simulink model "transientStability_R2013B_MDL"  (Simulink 8.2)
settings: Solver=ode4  SolverMode=SingleTasking  StartTime=0.0  StopTime=10  FixedStep=0.01  MaxStep=0.01  RelTol=1e-3  AbsTol=1e-2
undefined symbols (not defined in the file): j, mpc
(part 4 of 4)

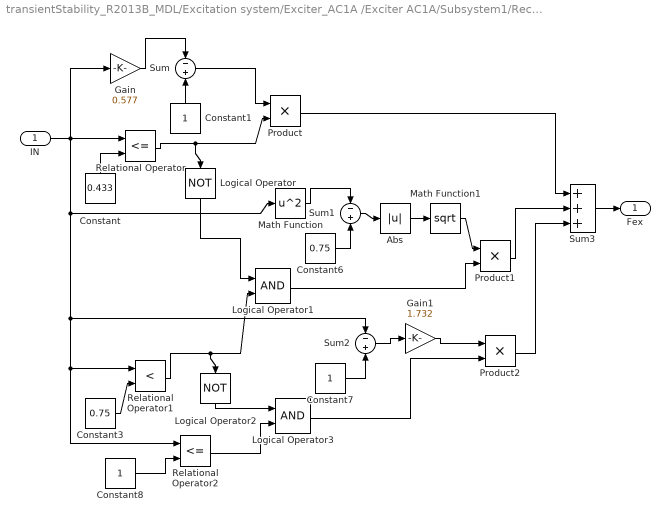
== system transientStability_R2013B_MDL/Excitation system/Exciter_AC1A /Exciter AC1A/Subsystem1/Rec-Reg Curve/Rec-Reg Eq  ==
  IN : Inport
  Abs : Abs  SaturateOnIntegerOverflow=on
  Constant : Constant  Value=0.433
  Constant1 : Constant
  Constant3 : Constant  Value=0.75
  Constant6 : Constant  Value=0.75
  Constant7 : Constant
  Constant8 : Constant
  Gain : Gain  Gain=0.577  SaturateOnIntegerOverflow=on  OutDataTypeStr=Inherit: Same as input  ParamDataTypeStr=Inherit: Same as input
  Gain1 : Gain  Gain=1.732  SaturateOnIntegerOverflow=on  OutDataTypeStr=Inherit: Same as input  ParamDataTypeStr=Inherit: Same as input
  Logical Operator : Logic  Operator=NOT
  Logical Operator1 : Logic
  Logical Operator2 : Logic  Operator=NOT
  Logical Operator3 : Logic
  Math Function : Math  Operator=square  SaturateOnIntegerOverflow=on
  Math Function1 : Math  Operator=sqrt  SaturateOnIntegerOverflow=on
  Product : Product  SaturateOnIntegerOverflow=on  RndMeth=Zero  InputSameDT=on  OutDataTypeStr=Inherit: Same as first input
  Product1 : Product  SaturateOnIntegerOverflow=on  RndMeth=Zero  InputSameDT=on  OutDataTypeStr=Inherit: Same as first input
  Product2 : Product  SaturateOnIntegerOverflow=on  RndMeth=Zero  InputSameDT=on  OutDataTypeStr=Inherit: Same as first input
  Relational Operator : RelationalOperator  Operator=<=  InputSameDT=on
  Relational Operator1 : RelationalOperator  Operator=<  InputSameDT=on
  Relational Operator2 : RelationalOperator  Operator=<=  InputSameDT=on
  Sum : Sum  Inputs=-+  SaturateOnIntegerOverflow=on  InputSameDT=on  OutDataTypeStr=Inherit: Same as first input
  Sum1 : Sum  Inputs=-+  SaturateOnIntegerOverflow=on  InputSameDT=on  OutDataTypeStr=Inherit: Same as first input
  Sum2 : Sum  Inputs=-+  SaturateOnIntegerOverflow=on  InputSameDT=on  OutDataTypeStr=Inherit: Same as first input
  Sum3 : Sum  Inputs=+++  SaturateOnIntegerOverflow=on  InputSameDT=on  OutDataTypeStr=Inherit: Same as first input
  Fex : Outport
  wires:
  Constant/1 -> Relational Operator/2
  Constant1/1 -> Sum/2
  Gain/1 -> Sum/1
  IN/1 -> Relational Operator/1, Gain/1, Math Function/1, Sum2/1, Relational Operator1/1, Relational Operator2/1
  Sum/1 -> Product/1
  Relational Operator/1 -> Product/2, Logical Operator/1
  Constant3/1 -> Relational Operator1/2
  Logical Operator/1 -> Logical Operator1/1
  Constant6/1 -> Sum1/2
  Math Function/1 -> Sum1/1
  Math Function1/1 -> Product1/1
  Logical Operator1/1 -> Product1/2
  Relational Operator1/1 -> Logical Operator1/2, Logical Operator2/1
  Constant7/1 -> Sum2/2
  Sum2/1 -> Gain1/1
  Gain1/1 -> Product2/1
  Constant8/1 -> Relational Operator2/2
  Logical Operator2/1 -> Logical Operator3/1
  Logical Operator3/1 -> Product2/2
  Product/1 -> Sum3/1
  Product1/1 -> Sum3/2
  Product2/1 -> Sum3/3
  Sum3/1 -> Fex/1
  Relational Operator2/1 -> Logical Operator3/2
  Sum1/1 -> Abs/1
  Abs/1 -> Math Function1/1

== system transientStability_R2013B_MDL/Excitation system/Exciter_AC1A /Exciter AC1A/Subsystem1/Saturation/Saturation ==
  VE : Inport
  Constant : Constant  Value=mpc.dynamicdata.gen_exciterParameters.AC1A_exciterParameters.B1
  Constant1 : Constant  Value=mpc.dynamicdata.gen_exciterParameters.AC1A_exciterParameters.A1
  Constant2 : Constant  Value=mpc.dynamicdata.gen_exciterParameters.AC1A_exciterParameters.KE_AC1A
  Math Function : Math  SaturateOnIntegerOverflow=on
  Product : Product  SaturateOnIntegerOverflow=on  RndMeth=Zero  InputSameDT=on  OutDataTypeStr=Inherit: Same as first input
  Product1 : Product  SaturateOnIntegerOverflow=on  RndMeth=Zero  InputSameDT=on  OutDataTypeStr=Inherit: Same as first input
  Product2 : Product  SaturateOnIntegerOverflow=on  RndMeth=Zero  InputSameDT=on  OutDataTypeStr=Inherit: Same as first input
  Sum2 : Sum  SaturateOnIntegerOverflow=on  InputSameDT=on  OutDataTypeStr=Inherit: Same as first input
  VRb : Outport
  wires:
  Constant/1 -> Product/1
  Product/1 -> Math Function/1
  Math Function/1 -> Product1/1
  Constant1/1 -> Product1/2
  Product1/1 -> Sum2/1
  Constant2/1 -> Sum2/2
  Sum2/1 -> Product2/1
  VE/1 -> Product/2, Product2/2
  Product2/1 -> VRb/1

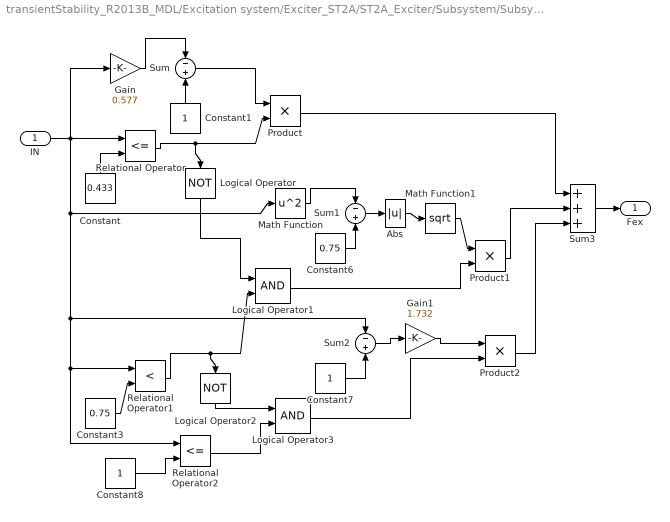
== system transientStability_R2013B_MDL/Excitation system/Exciter_ST2A/ST2A_Exciter/Subsystem/Subsystem2/Subsystem ==
  IN : Inport
  Abs : Abs  SaturateOnIntegerOverflow=on
  Constant : Constant  Value=0.433
  Constant1 : Constant
  Constant3 : Constant  Value=0.75
  Constant6 : Constant  Value=0.75
  Constant7 : Constant
  Constant8 : Constant
  Gain : Gain  Gain=0.577  SaturateOnIntegerOverflow=on  OutDataTypeStr=Inherit: Same as input  ParamDataTypeStr=Inherit: Same as input
  Gain1 : Gain  Gain=1.732  SaturateOnIntegerOverflow=on  OutDataTypeStr=Inherit: Same as input  ParamDataTypeStr=Inherit: Same as input
  Logical Operator : Logic  Operator=NOT
  Logical Operator1 : Logic
  Logical Operator2 : Logic  Operator=NOT
  Logical Operator3 : Logic
  Math Function : Math  Operator=square  SaturateOnIntegerOverflow=on
  Math Function1 : Math  Operator=sqrt  SaturateOnIntegerOverflow=on
  Product : Product  SaturateOnIntegerOverflow=on  RndMeth=Zero  InputSameDT=on  OutDataTypeStr=Inherit: Same as first input
  Product1 : Product  SaturateOnIntegerOverflow=on  RndMeth=Zero  InputSameDT=on  OutDataTypeStr=Inherit: Same as first input
  Product2 : Product  SaturateOnIntegerOverflow=on  RndMeth=Zero  InputSameDT=on  OutDataTypeStr=Inherit: Same as first input
  Relational Operator : RelationalOperator  Operator=<=  InputSameDT=on
  Relational Operator1 : RelationalOperator  Operator=<  InputSameDT=on
  Relational Operator2 : RelationalOperator  Operator=<=  InputSameDT=on
  Sum : Sum  Inputs=-+  SaturateOnIntegerOverflow=on  InputSameDT=on  OutDataTypeStr=Inherit: Same as first input
  Sum1 : Sum  Inputs=-+  SaturateOnIntegerOverflow=on  InputSameDT=on  OutDataTypeStr=Inherit: Same as first input
  Sum2 : Sum  Inputs=-+  SaturateOnIntegerOverflow=on  InputSameDT=on  OutDataTypeStr=Inherit: Same as first input
  Sum3 : Sum  Inputs=+++  SaturateOnIntegerOverflow=on  InputSameDT=on  OutDataTypeStr=Inherit: Same as first input
  Fex : Outport
  wires:
  Constant/1 -> Relational Operator/2
  Constant1/1 -> Sum/2
  Gain/1 -> Sum/1
  IN/1 -> Relational Operator/1, Gain/1, Math Function/1, Sum2/1, Relational Operator1/1, Relational Operator2/1
  Sum/1 -> Product/1
  Relational Operator/1 -> Product/2, Logical Operator/1
  Constant3/1 -> Relational Operator1/2
  Logical Operator/1 -> Logical Operator1/1
  Constant6/1 -> Sum1/2
  Math Function/1 -> Sum1/1
  Math Function1/1 -> Product1/1
  Logical Operator1/1 -> Product1/2
  Relational Operator1/1 -> Logical Operator1/2, Logical Operator2/1
  Constant7/1 -> Sum2/2
  Sum2/1 -> Gain1/1
  Gain1/1 -> Product2/1
  Constant8/1 -> Relational Operator2/2
  Logical Operator2/1 -> Logical Operator3/1
  Logical Operator3/1 -> Product2/2
  Product/1 -> Sum3/1
  Product1/1 -> Sum3/2
  Product2/1 -> Sum3/3
  Sum3/1 -> Fex/1
  Relational Operator2/1 -> Logical Operator3/2
  Sum1/1 -> Abs/1
  Abs/1 -> Math Function1/1
